simulink model "SF007A_SysFricLrng"  (R2013b)
settings: Solver=FixedStepDiscrete  SolverMode=SingleTasking  StartTime=0.0  StopTime=1  FixedStep=0.002  RelTol=1e-3
PostLoadFcn:
  | , if any(exist('dsrtsu_mdlpostloadfcn', 'file') == [2, 3, 6]), try dsrtsu_mdlpostloadfcn('Execute', bdroot); catch fprintf('Error in PostLoadFcn (dsrtsu_mdlpostloadfcn) for model "%s":\n %s\n', bdroot, lasterr); end, end,
undefined symbols (not defined in the file): ARCHGLBPRM_100MILLISEC_SEC_F32, ARCHGLBPRM_10MILLISEC_SEC_F32, ARCHGLBPRM_180OVERPI_ULS_F32, CONV100MICROSECTOSEC_ULS_F32, FLTINJ_SYSFRICLRNG_SYSFRICOFFS, FricLrngData, HiFricNtc, HWPTNUM_CNT_U08, HWPTNUMSUB1_CNT_U08, HWVELDECDIR_ULS_U08, HWVELINCDIR_ULS_U08, IDXCALCNSCAGFAC_ULS_U08, IDXSELN1_ULS_U08, IDXSELN2_ULS_U08, IDXSELN3_ULS_U08, LRNGENASCAFAC_MILLISEC_U32, NtcSts1, SCAGFACQUARTER_CNT_F32, SCAGFACTEN_CNT_U16, SECIDXSELN_ULS_U08, SysFricLrngBasLineEolFric, SysFricLrngBasLineFric, SysFricLrngBasLineHys, SysFricLrngBasLineRngCntr, SysFricLrngEolFricDifScagFac, SysFricLrngFricChgWght, SysFricLrngFricDiagcThd, SysFricLrngFricDiagcTiThd, SysFricLrngFricHysHwAgPt, SysFricLrngGain, SysFricLrngHwPosnAuthyThd, SysFricLrngHwVelConstrLim, SysFricLrngHwVelHiLim, SysFricLrngHwVelLoLim, SysFricLrngIgnCycFricChgLim, SysFricLrngLatAHiLim, SysFricLrngLatALoLim, SysFricLrngMaskVehSpd, SysFricLrngOperMod1, SysFricLrngRngCntrThd, SysFricLrngThd, SysFricLrngTHiLim, SysFricLrngTLoLim, SysFricLrngVehSpd, SYSFRICOFFSLIM_HWNWTMTR_F32, VEHSPDPTNUM1_ULS_U08, VEHSPDPTNUM2_ULS_U08
libraries: Fil x19, simulink x17, NxtrLim x10, NxtrAbslt x3, NxtrNvM x2, FixdToFloat x2, FloatToFixd x1, LnrIntrpn x1
(part 1 of 7)
settings Model: DSRTSU_INTERNAL_RTI_VER=370  DSRTSU_INTERNAL_RTI_TYPE=rti1401  Creator=fzv52m  LastModifiedBy=XZB1DB
settings Model: ModifiedHistory=|
  | Ver 004 Removed ignition latching of Friction Detection NTC to match software.
  | Limiting of P steps to one per ignition is being done with latching NTC allowing for the change
settings SolverCC: AutoInsertRateTranBlk=on  InsertRTBMode=Always
settings DataIOCC: LimitDataPoints=off  SaveFormat=Structure  ReturnWorkspaceOutputs=on
settings OptimizationCC: BlockReduction=off  InlineParams=on  ZeroExternalMemoryAtStartup=off  ZeroInternalMemoryAtStartup=off  OptimizeModelRefInitCode=on  LifeSpan=1
settings DebuggingCC: SignalInfNanChecking=error  SignalRangeChecking=warning  UnderspecifiedInitializationDetection=Simplified  SolverPrmCheckMsg=error  InheritedTsInSrcMsg=error  DiscreteInheritContinuousMsg=error  SingleTaskRateTransMsg=error  TasksWithSamePriorityMsg=error  SigSpecEnsureSampleTimeMsg=error  CheckMatrixSingularityMsg=error  ParameterUnderflowMsg=error  ParameterPrecisionLossMsg=error  ParameterTunabilityLossMsg=error  FixptConstUnderflowMsg=warning  FixptConstOverflowMsg=warning  VectorMatrixConversionMsg=error  SignalLabelMismatchMsg=error  UnconnectedInputMsg=error  UnconnectedOutputMsg=error  UnconnectedLineMsg=error  SFcnCompatibilityMsg=error  UniqueDataStoreMsg=warning  BusObjectLabelMismatch=error  RootOutportRequireBusObject=error  AssertControl=DisableAll  ModelReferenceIOMsg=error  ModelReferenceVersionMismatchMessage=warning  ModelReferenceIOMismatchMessage=error  ModelReferenceCSMismatchMessage=warning  ModelReferenceDataLoggingMessage=error  StateNameClashWarn=warning  StrictBusMsg=ErrorOnBusTreatedAsVector  NonBusSignalsTreatedAsBus=error  SFUnexpectedBacktrackingDiag=error  SFInvalidInputDataAccessInChartInitDiag=error  SFNoUnconditionalDefaultTransitionDiag=error  SFTransitionOutsideNaturalParentDiag=error  SFUnconditionalTransitionShadowingDiag=error  SFUndirectedBroadcastEventsDiag=error
settings ModelReferenceCC: ModelReferenceNumInstancesAllowed=Single
settings SFSimCC: SimGenImportedTypeDefs=on
settings RTWCC: SystemTargetFile=autosar.tlc  GenCodeOnly=on  TemplateMakefile=ert_default_tmf  Description=AUTOSAR  GenerateReport=on  ProcessScript=autosar_make_rtw_hook  LaunchReport=on
settings CodeAppCC: GenerateComments=off  IgnoreCustomStorageClasses=off  CustomSymbolStrType=$N$R$M  CustomSymbolStrBlkIO=$N$M  SimulinkBlockComments=off
settings STFCustomTargetCC: ParMdlRefBuildCompliant=on  CompOptLevelCompliant=on  IncludeMdlTerminateFcn=off  CombineOutputUpdateFcns=on  SuppressErrorStatus=on  ERTFirstTimeCompliant=on  ERTCustomFileBanners=on  SupportNonFinite=off  SupportComplex=off  SupportContinuousTime=off  SupportNonInlinedSFcns=off  MATLABClassNameForMDSCustomization=Simulink.SoftwareTarget.ERTCustomization  AutosarCompliant=on  GRTInterface=off  SystemTargetFile=autosar.tlc
settings ERTTargetCC: CodeReplacementLibrary=ANSI_C  ConcurrentExecutionCompliant=off  IncludeMdlTerminateFcn=off  SuppressErrorStatus=on  SupportNonFinite=off  SupportComplex=off  ModelStepFunctionPrototypeControlCompliant=off  CPPClassGenCompliant=off  AutosarCompliant=on  InlinedParameterPlacement=NonHierarchical  ERTCustomFileTemplate=example_file_process.tlc  EnableUserReplacementTypes=on

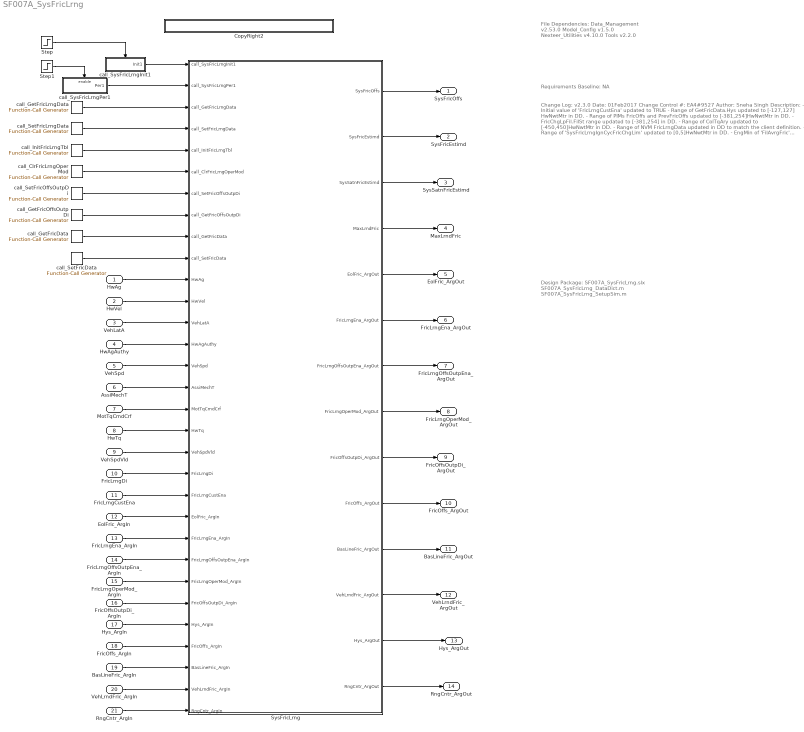
== system SF007A_SysFricLrng ==
  note: Requirements Baseline: NA
  note: File Dependencies:
      |
      | Data_Management v2.53.0
      | Model_Config v1.5.0
      | Nexteer_Utilities v4.10.0
      | Tools v2.2.0
  note: Change Log:
      |
      | v2.3.0
      | Date: 01Feb2017
      | Change Control #: EA4#9527
      | Author: Sneha Singh
      | Description:
      | - Initial value of 'FricLrngCustEna' updated to TRUE
      | - Range of GetFricData.Hys updated to [-127,127] HwNwtMtr in DD.
      | - Range of PIMs FricOffs and PrevFricOffs updated to [-381,254]HwNwtMtr in DD.
      | - FricChgLpFil.FilSt range updated to [-381,254] in DD.
      | - Range of ColTqAry updated to [-450,450]HwNwtMtr in DD.
      | - Range of NVM FricLrngData updated in DD to match the client definition.
      | - Range of 'SysFricLrngIgnCycFricChgLim' updated to [0,5]HwNwtMtr in DD.
      | - EngMin of 'FilAvrgFric' updated to -254 HwNwtMtr in DD.
      | - Range of 'SatnAvrgFric' updated to [-5,132]HwNwtMtr in DD.
      | - Definition of 'GetFricData' and 'SetFricData' updated in DD.
      | - Dimenions of NVM 'FricLrngData' updated in DD.
      | - Typecasting in the model has been updated to match source code.
      |
      | v2.2.0
      | Date: 29-NOV-2016
      | Change Control: EA4#8321
      | Function Owner:  Rangarajan Ramnujam
      | Description:
      | 1) Changes/clarification according to anomaly EA4#8103
      | 2) Added 'Get' and 'Set' client calls as per CR EA4#8418
      |
      |
      | v2.1.0
      | 1) Add output saturation for 'MaxLrndFric'
      | 2) Saturation constants added instead of using 'EngMin' and 'EngMax'
      |
      | v2.0.0
      | 1) Added extra output for Maximum Raw Average friction: Same friction value used for NTC diagnostic
      | 2)Else conditions added for LrngEna variable under path:
      | SF007A_SysFricLrng/SysFricLrng/SysFricLrngPer1/RunningAndCalibrationModes/RunningMode
      |
      | v1.4.0
      | 1) OR gate replaced with AND for LrngEna variable under path:
      | SF007A_SysFricLrng/SysFricLrng/SysFricLrngPer1/RunningAndCalibrationModes
      | 2) Logic updated under path
      | SF007A_SysFricLrng/SysFricLrng/SysFricLrngPer1/RunningAndCalibrationModes/Running Mode
      | 3) Eng min to -127 and Eng max to 254 updated for PIM 'FilAvrgFric' in Data Dict
      | 4) Logic for Indices calculation updated under below path. This change needed only in model as
      |     model uses one based Index logic. No code change required for this.
      |     SF007A_SysFricLrng/SysFricLrng/SysFricLrngPer1/RunningAndCalibrationModes/FricLearning/Indices Calculation
      | - Changes are highlighted in red. Code change needed for above mentioned changes 1, 2, and 4.
      |
      | v1.3.1
      | Date: 18-JULY-2016
      | Change Control: EA4#6450
      | DRW:  Hari Prasad(KPIT)
      | Description:
      | - Anomaly EA4#6361 Fixing for Gate variable look up table indexing.
      |   Removed 'Gate_Cnt_T_u08' temporary data store memory block.
      |   Logic related to it has been updated.
      | - Changes are highlighted in red. No code change needed.
      |
      | v1.3.0
      | Date: 07-APR-2016
      | Change Control #4835:
      | DRW:  Muragesh Asundi
      | Description:
      | - List of issues fixed are available under
      |   Doc/SF007_FDD_Issues.xlsx/Issues in V1.2.0
      | - In below path, Changed Gate from PIM to port inside subsystem
      |  as PIM wholds extra increment inside while loop
      |   SF007A_SysFricLrng/SysFricLrng/SysFricLrngPer1/RunningAndCalibrationModes/
      |   FricLearning/Range Counter Manager/Range Counter Control
      |
      | v1.2.0
      | Date: 30-Mar-2016
      | Change Control #4835:
      | DR W:  Muragesh Asundi
      | Description:
      | - List of issues fixed are available under
      |   Doc/SF007_FDD_Issues.xlsx/Issues in V1.1.0
      | - 'SetFricLrngOperMod' renamed to 'SetFricLrngData'
      | - 'SetEolFric' removed and merged with 'SetFricLrngData'
      | - Following PIMs have been removed from model and DD
      | 'HwAgPrev', 'HwVelPrev', 'ColTq'
      | - Monotony of callibration table 'SysFricLrngFricHysHwAgPt'
      | changed to 'Strictly_Increasing'
      | - Init value of PIM 'TotCntr' changed to 1
      |
      | v1.1.0
      | Date: 25-Mar-2016
      | Change Control #4835:
      | DRW:  Hari Prasad
      | Description:
      | - List of issues fixed are available under
      |   Doc/SF007_FDD_Issues.xlsx
      | - Changes are highlighed in red color
      |
      | v1.0.0
      | Date: 11-Mar-2016
      | Change Control #2719:
      | DRW:  Hari Prasad, Muragesh Asundi
      | Description:
      | - Initial Release of EA4 from EA3 V008
  note: Design Package:
      |
      | SF007A_SysFricLrng.slx
      | SF007A_SysFricLrng_DataDict.m
      | SF007A_SysFricLrng_SetupSim.m
  HwAg : Inport
  HwVel : Inport  Port=2
  VehLatA : Inport  Port=3
  HwAgAuthy : Inport  Port=4
  VehSpd : Inport  Port=5
  AssiMechT : Inport  Port=6
  MotTqCmdCrf : Inport  Port=7
  HwTq : Inport  Port=8
  VehSpdVld : Inport  Port=9
  FricLrngDi : Inport  Port=10
  FricLrngCustEna : Inport  Port=11
  EolFric_ArgIn : Inport  Port=12
  FricLrngEna_ArgIn : Inport  Port=13
  FricLrngOffsOutpEna_ArgIn : Inport  Port=14
  FricLrngOperMod_ArgIn : Inport  Port=15
  FricOffsOutpDi_ArgIn : Inport  Port=16
  Hys_ArgIn : Inport  Port=17
  FricOffs_ArgIn : Inport  Port=18
  BasLineFric_ArgIn : Inport  Port=19
  VehLrndFric_ArgIn : Inport  Port=20
  RngCntr_ArgIn : Inport  Port=21
  CopyRight2 : Subsystem  Description=|  mask(Copyright Information){none=on}
      | Copyright info block.                                               
      |                                                                     
      | Place copyright information at the top of every subsystem in design.
      mask prompts: none "No parameters"
      mask help: Place copyright information at the top of every subsystem in design.
      mask Display:
      | NxtrConf = 'Nexteer Confidential';
      | 
      | sys = bdroot; %handle for the current model ("system")
      | first = get_param(sys,'Created');
      | first = first(end-3:end);  %year is last four digits
      | 
      | last = get_param(sys,'LastModifiedDate');
      | if isempty(last)
      |     last = datestr(now,'yyyy');
      | else
      |     last = last(end-3:end);
      | end
      | 
      | if strcmp(first,last)
      |     fprintf('%s -- Copyright %s Nexteer',NxtrConf,first)
      | else
      |     fprintf('%s -- %s%s- %s Nexteer',NxtrConf,char(169),first,last)
      | end
  Step : Step  Before=1  After=0  SampleTime=0.010
  Step1 : Step  SampleTime=0.010
  SysFricLrng : Subsystem
  call_ClrFricLrngOperMod : simulink/Ports & Subsystems/Function-Call Generator  sample_time=0.010  numberOfIterations=1
  call_GetFricData : simulink/Ports & Subsystems/Function-Call Generator  sample_time=0.010  numberOfIterations=1
  call_GetFricLrngData : simulink/Ports & Subsystems/Function-Call Generator  sample_time=0.010  numberOfIterations=1
  call_GetFricOffsOutpDi : simulink/Ports & Subsystems/Function-Call Generator  sample_time=0.010  numberOfIterations=1
  call_InitFricLrngTbl : simulink/Ports & Subsystems/Function-Call Generator  sample_time=0.010  numberOfIterations=1
  call_SetFricData : simulink/Ports & Subsystems/Function-Call Generator  sample_time=0.010  numberOfIterations=1
  call_SetFricLrngData : simulink/Ports & Subsystems/Function-Call Generator  sample_time=0.010  numberOfIterations=1
  call_SetFricOffsOutpDi : simulink/Ports & Subsystems/Function-Call Generator  sample_time=0.010  numberOfIterations=1
  call_SysFricLrngInit1 : Subsystem  TreatAsAtomicUnit=on
  call_SysFricLrngPer1 : Subsystem  TreatAsAtomicUnit=on
  SysFricOffs : Outport
  SysFricEstimd : Outport  Port=2
  SysSatnFricEstimd : Outport  Port=3
  MaxLrndFric : Outport  Port=4
  EolFric_ArgOut : Outport  Port=5
  FricLrngEna_ArgOut : Outport  Port=6
  FricLrngOffsOutpEna_ArgOut : Outport  Port=7
  FricLrngOperMod_ArgOut : Outport  Port=8
  FricOffsOutpDi_ArgOut : Outport  Port=9
  FricOffs_ArgOut : Outport  Port=10
  BasLineFric_ArgOut : Outport  Port=11
  VehLrndFric_ArgOut : Outport  Port=12
  Hys_ArgOut : Outport  Port=13
  RngCntr_ArgOut : Outport  Port=14
  wires:
  MotTqCmdCrf/1 -> SysFricLrng/17(MotTqCmdCrf)
  FricLrngDi/1 -> SysFricLrng/20(FricLrngDi)
  HwVel/1 -> SysFricLrng/12(HwVel)
  HwAg/1 -> SysFricLrng/11(HwAg)
  HwTq/1 -> SysFricLrng/18(HwTq)
  VehSpdVld/1 -> SysFricLrng/19(VehSpdVld)
  call_GetFricLrngData/1 -> SysFricLrng/3(call_GetFricLrngData)
  HwAgAuthy/1 -> SysFricLrng/14(HwAgAuthy)
  AssiMechT/1 -> SysFricLrng/16(AssiMechT)
  VehLatA/1 -> SysFricLrng/13(VehLatA)
  VehSpd/1 -> SysFricLrng/15(VehSpd)
  SysFricLrng/1(SysFricOffs) -> SysFricOffs/1
  SysFricLrng/3(SysSatnFricEstimd) -> SysSatnFricEstimd/1
  SysFricLrng/2(SysFricEstimd) -> SysFricEstimd/1
  FricLrngCustEna/1 -> SysFricLrng/21(FricLrngCustEna)
  call_SetFricLrngData/1 -> SysFricLrng/4(call_SetFricLrngData)
  call_InitFricLrngTbl/1 -> SysFricLrng/5(call_InitFricLrngTbl)
  call_SetFricOffsOutpDi/1 -> SysFricLrng/7(call_SetFricOffsOutpDi)
  call_GetFricOffsOutpDi/1 -> SysFricLrng/8(call_GetFricOffsOutpDi)
  call_ClrFricLrngOperMod/1 -> SysFricLrng/6(call_ClrFricLrngOperMod)
  SysFricLrng/6(FricLrngEna_ArgOut) -> FricLrngEna_ArgOut/1
  SysFricLrng/8(FricLrngOperMod_ArgOut) -> FricLrngOperMod_ArgOut/1
  SysFricLrng/7(FricLrngOffsOutpEna_ArgOut) -> FricLrngOffsOutpEna_ArgOut/1
  SysFricLrng/9(FricOffsOutpDi_ArgOut) -> FricOffsOutpDi_ArgOut/1
  SysFricLrng/5(EolFric_ArgOut) -> EolFric_ArgOut/1
  FricLrngEna_ArgIn/1 -> SysFricLrng/23(FricLrngEna_ArgIn)
  FricLrngOffsOutpEna_ArgIn/1 -> SysFricLrng/24(FricLrngOffsOutpEna_ArgIn)
  FricLrngOperMod_ArgIn/1 -> SysFricLrng/25(FricLrngOperMod_ArgIn)
  EolFric_ArgIn/1 -> SysFricLrng/22(EolFric_ArgIn)
  FricOffsOutpDi_ArgIn/1 -> SysFricLrng/26(FricOffsOutpDi_ArgIn)
  call_SysFricLrngInit1/1(Init1) -> SysFricLrng/1(call_SysFricLrngInit1)
  Step/1 -> call_SysFricLrngInit1/Enable
  call_SysFricLrngPer1/1(Per1) -> SysFricLrng/2(call_SysFricLrngPer1)
  Step1/1 -> call_SysFricLrngPer1/Enable
  SysFricLrng/4(MaxLrndFric) -> MaxLrndFric/1
  SysFricLrng/10(FricOffs_ArgOut) -> FricOffs_ArgOut/1
  SysFricLrng/13(Hys_ArgOut) -> Hys_ArgOut/1
  SysFricLrng/11(BasLineFric_ArgOut) -> BasLineFric_ArgOut/1
  SysFricLrng/14(RngCntr_ArgOut) -> RngCntr_ArgOut/1
  SysFricLrng/12(VehLrndFric_ArgOut) -> VehLrndFric_ArgOut/1
  call_SetFricData/1 -> SysFricLrng/10(call_SetFricData)
  call_GetFricData/1 -> SysFricLrng/9(call_GetFricData)
  FricOffs_ArgIn/1 -> SysFricLrng/28(FricOffs_ArgIn)
  VehLrndFric_ArgIn/1 -> SysFricLrng/30(VehLrndFric_ArgIn)
  BasLineFric_ArgIn/1 -> SysFricLrng/29(BasLineFric_ArgIn)
  RngCntr_ArgIn/1 -> SysFricLrng/31(RngCntr_ArgIn)
  Hys_ArgIn/1 -> SysFricLrng/27(Hys_ArgIn)

== system SF007A_SysFricLrng/CopyRight2 ==

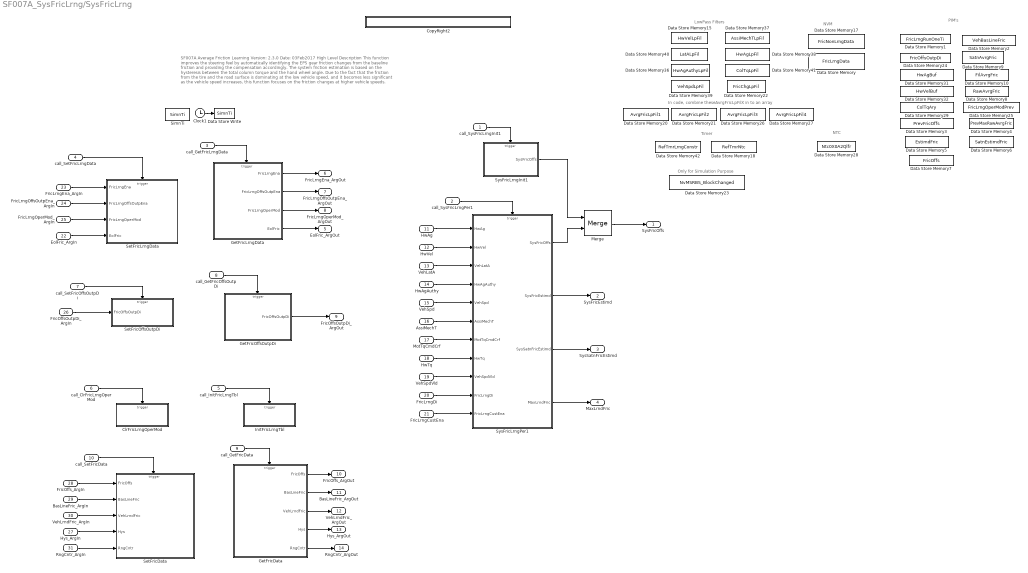
== system SF007A_SysFricLrng/SysFricLrng ==
  note: In code, combine theseAvrgFricLpFilX in to an array
  note: Only for Simulation Purpose
  note: PIM's
  note: Timer
  note: LowPass Filters
  note: NVM
  note: SF007A  Average Friction Learning
      | Version: 2.3.0          																															 					Date: 03Feb2017
      |
      | High Level Description
      |
      | This function improves the steering feel by automatically identifying the EPS gear friction changes from the baseline friction and providing the compensation accordingly. The system friction estimation
      |  is based on the hysteresis between the total column torque and the hand wheel angle. Due to the fact that the friction from the tire and the road surface is dominating at the low vehicle speed,  and it
      | becomes less significant as the vehicle speed increases, this function focuses on the friction changes at higher vehicle speeds.
  note: NTC
  call_SysFricLrngInit1 : Inport
  call_SysFricLrngPer1 : Inport  Port=2
  call_GetFricLrngData : Inport  Port=3
  call_SetFricLrngData : Inport  Port=4
  call_InitFricLrngTbl : Inport  Port=5
  call_ClrFricLrngOperMod : Inport  Port=6
  call_SetFricOffsOutpDi : Inport  Port=7
  call_GetFricOffsOutpDi : Inport  Port=8
  call_GetFricData : Inport  Port=9
  call_SetFricData : Inport  Port=10
  HwAg : Inport  Port=11
  HwVel : Inport  Port=12
  VehLatA : Inport  Port=13
  HwAgAuthy : Inport  Port=14
  VehSpd : Inport  Port=15
  AssiMechT : Inport  Port=16
  MotTqCmdCrf : Inport  Port=17
  HwTq : Inport  Port=18
  VehSpdVld : Inport  Port=19
  FricLrngDi : Inport  Port=20
  FricLrngCustEna : Inport  Port=21
  EolFric_ArgIn : Inport  Port=22
  FricLrngEna_ArgIn : Inport  Port=23
  FricLrngOffsOutpEna_ArgIn : Inport  Port=24
  FricLrngOperMod_ArgIn : Inport  Port=25
  FricOffsOutpDi_ArgIn : Inport  Port=26
  Hys_ArgIn : Inport  Port=27
  FricOffs_ArgIn : Inport  Port=28
  BasLineFric_ArgIn : Inport  Port=29
  VehLrndFric_ArgIn : Inport  Port=30
  RngCntr_ArgIn : Inport  Port=31
  Clock1 : Clock
  ClrFricLrngOperMod : Subsystem
  CopyRight2 : Subsystem  Description=|  mask(Copyright Information){none=on}
      | Copyright info block.                                               
      |                                                                     
      | Place copyright information at the top of every subsystem in design.
      mask prompts: none "No parameters"
      mask help: Place copyright information at the top of every subsystem in design.
      mask Display:
      | NxtrConf = 'Nexteer Confidential';
      | 
      | sys = bdroot; %handle for the current model ("system")
      | first = get_param(sys,'Created');
      | if(isempty(first))
      |     first = datestr(now,'yyyy');
      | else
      |     first = first(end-3:end);  %year is last four digits
      | end
      | 
      | last = get_param(sys,'LastModifiedDate');
      | if isempty(last)
      |     last = datestr(now,'yyyy');
      | else
      |     last = last(end-3:end);
      | end
      | 
      | if strcmp(first,last)
      |     fprintf('%s -- Copyright %s Nexteer',NxtrConf,first)
      | else
      |     fprintf('%s -- %s%s- %s Nexteer',NxtrConf,char(169),first,last)
      | end
  Data Store Memory : DataStoreMemory  DataStoreName=FricLrngData  InitialValue=[]  OutDataTypeStr=Bus: SysFricDataRec1  StateMustResolveToSignalObject=on
  Data Store Memory1 : DataStoreMemory  DataStoreName=FricLrngRunOneTi  StateMustResolveToSignalObject=on
  Data Store Memory10 : DataStoreMemory  DataStoreName=FilAvrgFric  InitialValue=[0 0 0 0]  OutDataTypeStr=single  StateMustResolveToSignalObject=on
  Data Store Memory15 : DataStoreMemory  DataStoreName=HwVelLpFil  InitialValue=struct('FilSt',single(0),'FilGain',single(0))  OutDataTypeStr=Bus: FilLpRec1  StateMustResolveToSignalObject=on
  Data Store Memory17 : DataStoreMemory  DataStoreName=FricNonLrngData  InitialValue=[]  OutDataTypeStr=Bus: SysFricNonLrngDataRec1  StateMustResolveToSignalObject=on
  Data Store Memory18 : DataStoreMemory  DataStoreName=RefTmrNtc  StateMustResolveToSignalObject=on
  Data Store Memory2 : DataStoreMemory  DataStoreName=VehBasLineFric  InitialValue=[0 0 0 0]  StateMustResolveToSignalObject=on
  Data Store Memory20 : DataStoreMemory  DataStoreName=AvrgFricLpFil1  InitialValue=struct('FilSt',single(0),'FilGain',single(0))  OutDataTypeStr=Bus: FilLpRec1  StateMustResolveToSignalObject=on
  Data Store Memory21 : DataStoreMemory  DataStoreName=AvrgFricLpFil2  InitialValue=struct('FilSt',single(0),'FilGain',single(0))  OutDataTypeStr=Bus: FilLpRec1  StateMustResolveToSignalObject=on
  Data Store Memory22 : DataStoreMemory  DataStoreName=FricChgLpFil  InitialValue=struct('FilSt',single(0),'FilGain',single(0))  OutDataTypeStr=Bus: FilLpRec1  StateMustResolveToSignalObject=on
  Data Store Memory23 : DataStoreMemory  DataStoreName=NvMSRBS_BlockChanged
  Data Store Memory24 : DataStoreMemory  DataStoreName=FricOffsOutpDi  StateMustResolveToSignalObject=on
  Data Store Memory25 : DataStoreMemory  DataStoreName=FricLrngOperModPrev  InitialValue=[]  StateMustResolveToSignalObject=on
  Data Store Memory26 : DataStoreMemory  DataStoreName=AvrgFricLpFil3  InitialValue=struct('FilSt',single(0),'FilGain',single(0))  OutDataTypeStr=Bus: FilLpRec1  StateMustResolveToSignalObject=on
  Data Store Memory27 : DataStoreMemory  DataStoreName=AvrgFricLpFil4  InitialValue=struct('FilSt',single(0),'FilGain',single(0))  OutDataTypeStr=Bus: FilLpRec1  StateMustResolveToSignalObject=on
  Data Store Memory28 : DataStoreMemory  DataStoreName=Ntc0X0A2Qlfr  InitialValue=SigQlfr1.SIGQLFR_NORES
  Data Store Memory29 : DataStoreMemory  DataStoreName=ColTqAry  InitialValue=[]  StateMustResolveToSignalObject=on
  Data Store Memory3 : DataStoreMemory  DataStoreName=PrevFricOffs  InitialValue=[]  StateMustResolveToSignalObject=on
  Data Store Memory31 : DataStoreMemory  DataStoreName=HwAgBuf  InitialValue=[0 0 0 0 0 0 0 0 0 0 0 0]  StateMustResolveToSignalObject=on
  Data Store Memory32 : DataStoreMemory  DataStoreName=HwVelBuf  InitialValue=[0 0 0 0 0 0 0 0 0 0 0 0]  StateMustResolveToSignalObject=on
  Data Store Memory36 : DataStoreMemory  DataStoreName=HwAgAuthyLpFil  InitialValue=struct('FilSt',single(0),'FilGain',single(0))  OutDataTypeStr=Bus: FilLpRec1  StateMustResolveToSignalObject=on
  Data Store Memory37 : DataStoreMemory  DataStoreName=AssiMechTLpFil  InitialValue=struct('FilSt',single(0),'FilGain',single(0))  OutDataTypeStr=Bus: FilLpRec1  StateMustResolveToSignalObject=on
  Data Store Memory38 : DataStoreMemory  DataStoreName=HwAgLpFil  InitialValue=struct('FilSt',single(0),'FilGain',single(0))  OutDataTypeStr=Bus: FilLpRec1  StateMustResolveToSignalObject=on
  Data Store Memory39 : DataStoreMemory  DataStoreName=VehSpdLpFil  InitialValue=struct('FilSt',single(0),'FilGain',single(0))  OutDataTypeStr=Bus: FilLpRec1  StateMustResolveToSignalObject=on
  Data Store Memory4 : DataStoreMemory  DataStoreName=PrevMaxRawAvrgFric  InitialValue=[]  OutDataTypeStr=single  StateMustResolveToSignalObject=on
  Data Store Memory40 : DataStoreMemory  DataStoreName=LatALpFil  InitialValue=struct('FilSt',single(0),'FilGain',single(0))  OutDataTypeStr=Bus: FilLpRec1  StateMustResolveToSignalObject=on
  Data Store Memory41 : DataStoreMemory  DataStoreName=ColTqLpFil  InitialValue=struct('FilSt',single(0),'FilGain',single(0))  OutDataTypeStr=Bus: FilLpRec1  StateMustResolveToSignalObject=on
  Data Store Memory42 : DataStoreMemory  DataStoreName=RefTmrLrngConstr  StateMustResolveToSignalObject=on
  Data Store Memory5 : DataStoreMemory  DataStoreName=EstimdFric  InitialValue=[]  OutDataTypeStr=single  StateMustResolveToSignalObject=on
  Data Store Memory6 : DataStoreMemory  DataStoreName=SatnEstimdFric  InitialValue=[]  OutDataTypeStr=single  StateMustResolveToSignalObject=on
  Data Store Memory7 : DataStoreMemory  DataStoreName=FricOffs  InitialValue=[]  OutDataTypeStr=single  StateMustResolveToSignalObject=on
  Data Store Memory8 : DataStoreMemory  DataStoreName=RawAvrgFric  InitialValue=[0 0 0 0]  OutDataTypeStr=single  StateMustResolveToSignalObject=on
  Data Store Memory9 : DataStoreMemory  DataStoreName=SatnAvrgFric  InitialValue=[0 0 0 0]  StateMustResolveToSignalObject=on
  Data Store Write : DataStoreWrite  DataStoreName=SimnTi
  GetFricData : Subsystem
  GetFricLrngData : Subsystem
  GetFricOffsOutpDi : Subsystem
  InitFricLrngTbl : Subsystem
  Merge : Merge
  SetFricData : Subsystem
  SetFricLrngData : Subsystem
  SetFricOffsOutpDi : Subsystem
  SimnTi : DataStoreMemory  DataStoreName=SimnTi
  SysFricLrngInit1 : Subsystem
  SysFricLrngPer1 : Subsystem
  SysFricOffs : Outport
  SysFricEstimd : Outport  Port=2
  SysSatnFricEstimd : Outport  Port=3
  MaxLrndFric : Outport  Port=4
  EolFric_ArgOut : Outport  Port=5
  FricLrngEna_ArgOut : Outport  Port=6
  FricLrngOffsOutpEna_ArgOut : Outport  Port=7
  FricLrngOperMod_ArgOut : Outport  Port=8
  FricOffsOutpDi_ArgOut : Outport  Port=9
  FricOffs_ArgOut : Outport  Port=10
  BasLineFric_ArgOut : Outport  Port=11
  VehLrndFric_ArgOut : Outport  Port=12
  Hys_ArgOut : Outport  Port=13
  RngCntr_ArgOut : Outport  Port=14
  wires:
  call_SysFricLrngInit1/1 -> SysFricLrngInit1/Trigger
  HwAg/1 -> SysFricLrngPer1/1(HwAg)
  HwVel/1 -> SysFricLrngPer1/2(HwVel)
  VehLatA/1 -> SysFricLrngPer1/3(VehLatA)
  HwAgAuthy/1 -> SysFricLrngPer1/4(HwAgAuthy)
  VehSpd/1 -> SysFricLrngPer1/5(VehSpd)
  AssiMechT/1 -> SysFricLrngPer1/6(AssiMechT)
  MotTqCmdCrf/1 -> SysFricLrngPer1/7(MotTqCmdCrf)
  HwTq/1 -> SysFricLrngPer1/8(HwTq)
  VehSpdVld/1 -> SysFricLrngPer1/9(VehSpdVld)
  FricLrngDi/1 -> SysFricLrngPer1/10(FricLrngDi)
  call_SysFricLrngPer1/1 -> SysFricLrngPer1/Trigger
  Clock1/1 -> Data Store Write/1
  SysFricLrngPer1/3(SysSatnFricEstimd) -> SysSatnFricEstimd/1
  SysFricLrngPer1/2(SysFricEstimd) -> SysFricEstimd/1
  FricLrngCustEna/1 -> SysFricLrngPer1/11(FricLrngCustEna)
  call_SetFricLrngData/1 -> SetFricLrngData/Trigger
  call_GetFricLrngData/1 -> GetFricLrngData/Trigger
  call_SetFricOffsOutpDi/1 -> SetFricOffsOutpDi/Trigger
  call_GetFricOffsOutpDi/1 -> GetFricOffsOutpDi/Trigger
  call_InitFricLrngTbl/1 -> InitFricLrngTbl/Trigger
  call_ClrFricLrngOperMod/1 -> ClrFricLrngOperMod/Trigger
  GetFricLrngData/1(FricLrngEna) -> FricLrngEna_ArgOut/1
  GetFricLrngData/3(FricLrngOperMod) -> FricLrngOperMod_ArgOut/1
  GetFricLrngData/2(FricLrngOffsOutpEna) -> FricLrngOffsOutpEna_ArgOut/1
  FricLrngEna_ArgIn/1 -> SetFricLrngData/1(FricLrngEna)
  FricLrngOperMod_ArgIn/1 -> SetFricLrngData/3(FricLrngOperMod)
  FricLrngOffsOutpEna_ArgIn/1 -> SetFricLrngData/2(FricLrngOffsOutpEna)
  FricOffsOutpDi_ArgIn/1 -> SetFricOffsOutpDi/1(FricOffsOutpDi)
  GetFricOffsOutpDi/1(FricOffsOutpDi) -> FricOffsOutpDi_ArgOut/1
  GetFricLrngData/4(EolFric) -> EolFric_ArgOut/1
  SysFricLrngInit1/1(SysFricOffs) -> Merge/1
  SysFricLrngPer1/1(SysFricOffs) -> Merge/2
  Merge/1 -> SysFricOffs/1
  EolFric_ArgIn/1 -> SetFricLrngData/4(EolFric)
  SysFricLrngPer1/4(MaxLrndFric) -> MaxLrndFric/1
  call_SetFricData/1 -> SetFricData/Trigger
  call_GetFricData/1 -> GetFricData/Trigger
  FricOffs_ArgIn/1 -> SetFricData/1(FricOffs)
  VehLrndFric_ArgIn/1 -> SetFricData/3(VehLrndFric)
  BasLineFric_ArgIn/1 -> SetFricData/2(BasLineFric)
  RngCntr_ArgIn/1 -> SetFricData/5(RngCntr)
  GetFricData/1(FricOffs) -> FricOffs_ArgOut/1
  GetFricData/4(Hys) -> Hys_ArgOut/1
  GetFricData/2(BasLineFric) -> BasLineFric_ArgOut/1
  GetFricData/5(RngCntr) -> RngCntr_ArgOut/1
  GetFricData/3(VehLrndFric) -> VehLrndFric_ArgOut/1
  Hys_ArgIn/1 -> SetFricData/4(Hys)

== system SF007A_SysFricLrng/call_SysFricLrngInit1 ==
  Enable : EnablePort
  CopyRight2 : Subsystem  Description=|  mask(Copyright Information){none=on}
      | Copyright info block.                                               
      |                                                                     
      | Place copyright information at the top of every subsystem in design.
      mask prompts: none "No parameters"
      mask help: Place copyright information at the top of every subsystem in design.
      mask Display:
      | NxtrConf = 'Nexteer Confidential';
      | 
      | sys = bdroot; %handle for the current model ("system")
      | first = get_param(sys,'Created');
      | if(isempty(first))
      |     first = datestr(now,'yyyy');
      | else
      |     first = first(end-3:end);  %year is last four digits
      | end
      | 
      | last = get_param(sys,'LastModifiedDate');
      | if isempty(last)
      |     last = datestr(now,'yyyy');
      | else
      |     last = last(end-3:end);
      | end
      | 
      | if strcmp(first,last)
      |     fprintf('%s -- Copyright %s Nexteer',NxtrConf,first)
      | else
      |     fprintf('%s -- %s%s- %s Nexteer',NxtrConf,char(169),first,last)
      | end
  Function-Call Generator : simulink/Ports & Subsystems/Function-Call Generator  sample_time=.01  numberOfIterations=1
  Init1 : Outport
  wires:
  Function-Call Generator/1 -> Init1/1

== system SF007A_SysFricLrng/call_SysFricLrngPer1 ==
  Enable : EnablePort
  CopyRight2 : Subsystem  Description=|  mask(Copyright Information){none=on}
      | Copyright info block.                                               
      |                                                                     
      | Place copyright information at the top of every subsystem in design.
      mask prompts: none "No parameters"
      mask help: Place copyright information at the top of every subsystem in design.
      mask Display:
      | NxtrConf = 'Nexteer Confidential';
      | 
      | sys = bdroot; %handle for the current model ("system")
      | first = get_param(sys,'Created');
      | if(isempty(first))
      |     first = datestr(now,'yyyy');
      | else
      |     first = first(end-3:end);  %year is last four digits
      | end
      | 
      | last = get_param(sys,'LastModifiedDate');
      | if isempty(last)
      |     last = datestr(now,'yyyy');
      | else
      |     last = last(end-3:end);
      | end
      | 
      | if strcmp(first,last)
      |     fprintf('%s -- Copyright %s Nexteer',NxtrConf,first)
      | else
      |     fprintf('%s -- %s%s- %s Nexteer',NxtrConf,char(169),first,last)
      | end
  Function-Call Generator : simulink/Ports & Subsystems/Function-Call Generator  sample_time=.01  numberOfIterations=1
  Per1 : Outport
  wires:
  Function-Call Generator/1 -> Per1/1

== system SF007A_SysFricLrng/SysFricLrng/ClrFricLrngOperMod ==
  note: Set Ram Block Status for 'FricLrngData' moved to Init
  function : TriggerPort  TriggerType=function-call
  Constant1 : Constant  Value=false  OutDataTypeStr=boolean
      settings: AttributesFormatString=%<OutDataTypeStr>
  CopyRight2 : Subsystem  Description=|  mask(Copyright Information){none=on}
      | Copyright info block.                                               
      |                                                                     
      | Place copyright information at the top of every subsystem in design.
      mask prompts: none "No parameters"
      mask help: Place copyright information at the top of every subsystem in design.
      mask Display:
      | NxtrConf = 'Nexteer Confidential';
      | 
      | sys = bdroot; %handle for the current model ("system")
      | first = get_param(sys,'Created');
      | if(isempty(first))
      |     first = datestr(now,'yyyy');
      | else
      |     first = first(end-3:end);  %year is last four digits
      | end
      | 
      | last = get_param(sys,'LastModifiedDate');
      | if isempty(last)
      |     last = datestr(now,'yyyy');
      | else
      |     last = last(end-3:end);
      | end
      | 
      | if strcmp(first,last)
      |     fprintf('%s -- Copyright %s Nexteer',NxtrConf,first)
      | else
      |     fprintf('%s -- %s%s- %s Nexteer',NxtrConf,char(169),first,last)
      | end
  Data Store Read : DataStoreRead  DataStoreName=FricLrngData  DataStoreElements=FricLrngData.SysFricLrngOperMod
  Data Store Write : DataStoreWrite  DataStoreName=FricLrngOperModPrev
  Data Store Write1 : DataStoreWrite  DataStoreName=FricLrngData  DataStoreElements=FricLrngData.SysFricLrngOperMod
  Data Store Write2 : DataStoreWrite  DataStoreName=FricLrngRunOneTi
  Enumerated Constant : simulink/Sources/Enumerated Constant  OutDataTypeStr=Enum: SysFricLrngOperMod1  Value=SysFricLrngOperMod1.SYSFRICLRNGOPERMOD_CLEAR  SampleTime=inf
  wires:
  Constant1/1 -> Data Store Write2/1
  Enumerated Constant/1 -> Data Store Write1/1
  Data Store Read/1 -> Data Store Write/1

== system SF007A_SysFricLrng/SysFricLrng/CopyRight2 ==

== system SF007A_SysFricLrng/SysFricLrng/GetFricData ==
  note: Get NVM Data
  function : TriggerPort  TriggerType=function-call
  CopyRight2 : Subsystem  Description=|  mask(Copyright Information){none=on}
      | Copyright info block.                                               
      |                                                                     
      | Place copyright information at the top of every subsystem in design.
      mask prompts: none "No parameters"
      mask help: Place copyright information at the top of every subsystem in design.
      mask Display:
      | NxtrConf = 'Nexteer Confidential';
      | 
      | sys = bdroot; %handle for the current model ("system")
      | first = get_param(sys,'Created');
      | first = first(end-3:end);  %year is last four digits
      | 
      | last = get_param(sys,'LastModifiedDate');
      | if isempty(last)
      |     last = datestr(now,'yyyy');
      | else
      |     last = last(end-3:end);
      | end
      | 
      | if strcmp(first,last)
      |     fprintf('%s -- Copyright %s Nexteer',NxtrConf,first)
      | else
      |     fprintf('%s -- %s%s- %s Nexteer',NxtrConf,char(169),first,last)
      | end
  Data Store Read : DataStoreRead  DataStoreName=FricLrngData  DataStoreElements=FricLrngData.FricOffs#FricLrngData.BasLineFric(:,:)#FricLrngData.VehLrndFric(:,:)#FricLrngData.Hys(:,:)#FricLrngData.RngCntr(:,:)
  FricOffs : Outport
  BasLineFric : Outport  Port=2
  VehLrndFric : Outport  Port=3
  Hys : Outport  Port=4
  RngCntr : Outport  Port=5
  wires:
  Data Store Read/5 -> RngCntr/1
  Data Store Read/1 -> FricOffs/1
  Data Store Read/2 -> BasLineFric/1
  Data Store Read/3 -> VehLrndFric/1
  Data Store Read/4 -> Hys/1

== system SF007A_SysFricLrng/SysFricLrng/GetFricLrngData ==
  note: Get NVM Data
  function : TriggerPort  TriggerType=function-call
  CopyRight2 : Subsystem  Description=|  mask(Copyright Information){none=on}
      | Copyright info block.                                               
      |                                                                     
      | Place copyright information at the top of every subsystem in design.
      mask prompts: none "No parameters"
      mask help: Place copyright information at the top of every subsystem in design.
      mask Display:
      | NxtrConf = 'Nexteer Confidential';
      | 
      | sys = bdroot; %handle for the current model ("system")
      | first = get_param(sys,'Created');
      | first = first(end-3:end);  %year is last four digits
      | 
      | last = get_param(sys,'LastModifiedDate');
      | if isempty(last)
      |     last = datestr(now,'yyyy');
      | else
      |     last = last(end-3:end);
      | end
      | 
      | if strcmp(first,last)
      |     fprintf('%s -- Copyright %s Nexteer',NxtrConf,first)
      | else
      |     fprintf('%s -- %s%s- %s Nexteer',NxtrConf,char(169),first,last)
      | end
  Data Store Read : DataStoreRead  DataStoreName=FricLrngData  DataStoreElements=FricLrngData.SysFricLrngOperMod
  Data Store Read1 : DataStoreRead  DataStoreName=FricNonLrngData  DataStoreElements=FricNonLrngData.EnaFricLrng#FricNonLrngData.EnaFricOffsOutp#FricNonLrngData.EolFric
  FricLrngEna : Outport
  FricLrngOffsOutpEna : Outport  Port=2
  FricLrngOperMod : Outport  Port=3
  EolFric : Outport  Port=4
  wires:
  Data Store Read/1 -> FricLrngOperMod/1
  Data Store Read1/1 -> FricLrngEna/1
  Data Store Read1/2 -> FricLrngOffsOutpEna/1
  Data Store Read1/3 -> EolFric/1

== system SF007A_SysFricLrng/SysFricLrng/GetFricOffsOutpDi ==
  function : TriggerPort  TriggerType=function-call
  CopyRight2 : Subsystem  Description=|  mask(Copyright Information){none=on}
      | Copyright info block.                                               
      |                                                                     
      | Place copyright information at the top of every subsystem in design.
      mask prompts: none "No parameters"
      mask help: Place copyright information at the top of every subsystem in design.
      mask Display:
      | NxtrConf = 'Nexteer Confidential';
      | 
      | sys = bdroot; %handle for the current model ("system")
      | first = get_param(sys,'Created');
      | first = first(end-3:end);  %year is last four digits
      | 
      | last = get_param(sys,'LastModifiedDate');
      | if isempty(last)
      |     last = datestr(now,'yyyy');
      | else
      |     last = last(end-3:end);
      | end
      | 
      | if strcmp(first,last)
      |     fprintf('%s -- Copyright %s Nexteer',NxtrConf,first)
      | else
      |     fprintf('%s -- %s%s- %s Nexteer',NxtrConf,char(169),first,last)
      | end
  Data Store Read1 : DataStoreRead  DataStoreName=FricOffsOutpDi
  FricOffsOutpDi : Outport
  wires:
  Data Store Read1/1 -> FricOffsOutpDi/1

== system SF007A_SysFricLrng/SysFricLrng/InitFricLrngTbl ==
  note: Set Ram Block Status moved to Init
  function : TriggerPort  TriggerType=function-call
  Constant1 : Constant  Value=false  OutDataTypeStr=boolean
      settings: AttributesFormatString=%<OutDataTypeStr>
  CopyRight2 : Subsystem  Description=|  mask(Copyright Information){none=on}
      | Copyright info block.                                               
      |                                                                     
      | Place copyright information at the top of every subsystem in design.
      mask prompts: none "No parameters"
      mask help: Place copyright information at the top of every subsystem in design.
      mask Display:
      | NxtrConf = 'Nexteer Confidential';
      | 
      | sys = bdroot; %handle for the current model ("system")
      | first = get_param(sys,'Created');
      | if(isempty(first))
      |     first = datestr(now,'yyyy');
      | else
      |     first = first(end-3:end);  %year is last four digits
      | end
      | 
      | last = get_param(sys,'LastModifiedDate');
      | if isempty(last)
      |     last = datestr(now,'yyyy');
      | else
      |     last = last(end-3:end);
      | end
      | 
      | if strcmp(first,last)
      |     fprintf('%s -- Copyright %s Nexteer',NxtrConf,first)
      | else
      |     fprintf('%s -- %s%s- %s Nexteer',NxtrConf,char(169),first,last)
      | end
  Data Store Read : DataStoreRead  DataStoreName=FricLrngData  DataStoreElements=FricLrngData.SysFricLrngOperMod
  Data Store Write : DataStoreWrite  DataStoreName=FricLrngOperModPrev
  Data Store Write1 : DataStoreWrite  DataStoreName=FricLrngData  DataStoreElements=FricLrngData.SysFricLrngOperMod
  Data Store Write2 : DataStoreWrite  DataStoreName=FricLrngRunOneTi
  Enumerated Constant : simulink/Sources/Enumerated Constant  OutDataTypeStr=Enum: SysFricLrngOperMod1  Value=SysFricLrngOperMod1.SYSFRICLRNGOPERMOD_BASELINE  SampleTime=inf
  wires:
  Data Store Read/1 -> Data Store Write/1
  Enumerated Constant/1 -> Data Store Write1/1
  Constant1/1 -> Data Store Write2/1

== system SF007A_SysFricLrng/SysFricLrng/SetFricData ==
  note: Set Ram Block Status for 'FricLrngData' moved to Init
  note: update NVM
  FricOffs : Inport
  BasLineFric : Inport  Port=2
  VehLrndFric : Inport  Port=3
  Hys : Inport  Port=4
  RngCntr : Inport  Port=5
  function : TriggerPort  TriggerType=function-call
  CopyRight2 : Subsystem  Description=|  mask(Copyright Information){none=on}
      | Copyright info block.                                               
      |                                                                     
      | Place copyright information at the top of every subsystem in design.
      mask prompts: none "No parameters"
      mask help: Place copyright information at the top of every subsystem in design.
      mask Display:
      | NxtrConf = 'Nexteer Confidential';
      | 
      | sys = bdroot; %handle for the current model ("system")
      | first = get_param(sys,'Created');
      | first = first(end-3:end);  %year is last four digits
      | 
      | last = get_param(sys,'LastModifiedDate');
      | if isempty(last)
      |     last = datestr(now,'yyyy');
      | else
      |     last = last(end-3:end);
      | end
      | 
      | if strcmp(first,last)
      |     fprintf('%s -- Copyright %s Nexteer',NxtrConf,first)
      | else
      |     fprintf('%s -- %s%s- %s Nexteer',NxtrConf,char(169),first,last)
      | end
  Data Store Write3 : DataStoreWrite  DataStoreName=FricLrngData  DataStoreElements=FricLrngData.FricOffs#FricLrngData.BasLineFric(:,:)#FricLrngData.VehLrndFric(:,:)#FricLrngData.Hys(:,:)#FricLrngData.RngCntr(:,:)
  wires:
  Hys/1 -> Data Store Write3/4
  FricOffs/1 -> Data Store Write3/1
  BasLineFric/1 -> Data Store Write3/2
  VehLrndFric/1 -> Data Store Write3/3
  RngCntr/1 -> Data Store Write3/5

== system SF007A_SysFricLrng/SysFricLrng/SetFricLrngData ==
  note: Set Ram Block Status for 'FricLrngData' moved to Init
  note: update NVM
  FricLrngEna : Inport
  FricLrngOffsOutpEna : Inport  Port=2
  FricLrngOperMod : Inport  Port=3
  EolFric : Inport  Port=4
  function : TriggerPort  TriggerType=function-call
  Constant1 : Constant  Value=true  OutDataTypeStr=boolean
      settings: AttributesFormatString=%<OutDataTypeStr>
  CopyRight2 : Subsystem  Description=|  mask(Copyright Information){none=on}
      | Copyright info block.                                               
      |                                                                     
      | Place copyright information at the top of every subsystem in design.
      mask prompts: none "No parameters"
      mask help: Place copyright information at the top of every subsystem in design.
      mask Display:
      | NxtrConf = 'Nexteer Confidential';
      | 
      | sys = bdroot; %handle for the current model ("system")
      | first = get_param(sys,'Created');
      | first = first(end-3:end);  %year is last four digits
      | 
      | last = get_param(sys,'LastModifiedDate');
      | if isempty(last)
      |     last = datestr(now,'yyyy');
      | else
      |     last = last(end-3:end);
      | end
      | 
      | if strcmp(first,last)
      |     fprintf('%s -- Copyright %s Nexteer',NxtrConf,first)
      | else
      |     fprintf('%s -- %s%s- %s Nexteer',NxtrConf,char(169),first,last)
      | end
  Data Store Write : DataStoreWrite  DataStoreName=FricLrngOperModPrev
  Data Store Write1 : DataStoreWrite  DataStoreName=FricLrngData  DataStoreElements=FricLrngData.SysFricLrngOperMod
  Data Store Write3 : DataStoreWrite  DataStoreName=FricNonLrngData  DataStoreElements=FricNonLrngData.EnaFricLrng#FricNonLrngData.EnaFricOffsOutp#FricNonLrngData.EolFric
  Set Ram Block Status1 : NxtrNvM/Set Ram Block Status  FuncName=Set Ram Block Status  NvMBlockName=FricNonLrngData  VoidFuncRtn=on  BlockChanged_DSN=NvMSRBS_BlockChanged  Return_DSN=NvMSRBS_Return
      settings: AttributesFormatString=%<FuncName>
  wires:
  Constant1/1 -> Set Ram Block Status1/1
  FricLrngOperMod/1 -> Data Store Write/1, Data Store Write1/1
  FricLrngEna/1 -> Data Store Write3/1
  FricLrngOffsOutpEna/1 -> Data Store Write3/2
  EolFric/1 -> Data Store Write3/3

== system SF007A_SysFricLrng/SysFricLrng/SetFricOffsOutpDi ==
  FricOffsOutpDi : Inport
  function : TriggerPort  TriggerType=function-call
  CopyRight2 : Subsystem  Description=|  mask(Copyright Information){none=on}
      | Copyright info block.                                               
      |                                                                     
      | Place copyright information at the top of every subsystem in design.
      mask prompts: none "No parameters"
      mask help: Place copyright information at the top of every subsystem in design.
      mask Display:
      | NxtrConf = 'Nexteer Confidential';
      | 
      | sys = bdroot; %handle for the current model ("system")
      | first = get_param(sys,'Created');
      | first = first(end-3:end);  %year is last four digits
      | 
      | last = get_param(sys,'LastModifiedDate');
      | if isempty(last)
      |     last = datestr(now,'yyyy');
      | else
      |     last = last(end-3:end);
      | end
      | 
      | if strcmp(first,last)
      |     fprintf('%s -- Copyright %s Nexteer',NxtrConf,first)
      | else
      |     fprintf('%s -- %s%s- %s Nexteer',NxtrConf,char(169),first,last)
      | end
  Data Store Write : DataStoreWrite  DataStoreName=FricOffsOutpDi
  wires:
  FricOffsOutpDi/1 -> Data Store Write/1

== system SF007A_SysFricLrng/SysFricLrng/SysFricLrngInit1 ==
  note: Note: Removed comments as per anomaly fix to prevent confusion
  function : TriggerPort  TriggerType=function-call
  AssiMechTLpFil : Fil/FilLpInit  Ic=0  Ts=ARCHGLBPRM_10MILLISEC_SEC_F32  Freq=SysFricLrngDataPrepLpFilFrq  StVar=AssiMechTLpFil
  AvrgFricLpFil1 : Fil/FilLpInit  Ic=0  Ts=ARCHGLBPRM_10MILLISEC_SEC_F32  Freq=SysFricLrngAvrgFricFrq  StVar=AvrgFricLpFil1
  AvrgFricLpFil2 : Fil/FilLpInit  Ic=0  Ts=ARCHGLBPRM_10MILLISEC_SEC_F32  Freq=SysFricLrngAvrgFricFrq  StVar=AvrgFricLpFil2
  AvrgFricLpFil3 : Fil/FilLpInit  Ic=0  Ts=ARCHGLBPRM_10MILLISEC_SEC_F32  Freq=SysFricLrngAvrgFricFrq  StVar=AvrgFricLpFil3
  AvrgFricLpFil4 : Fil/FilLpInit  Ic=0  Ts=ARCHGLBPRM_10MILLISEC_SEC_F32  Freq=SysFricLrngAvrgFricFrq  StVar=AvrgFricLpFil4
  ColTqLpFil : Fil/FilLpInit  Ic=0  Ts=ARCHGLBPRM_10MILLISEC_SEC_F32  Freq=SysFricLrngDataPrepLpFilFrq  StVar=ColTqLpFil
  Constant : Constant  Value=VEHSPDPTNUM1_ULS_U08
  Constant1 : Constant  Value=true  OutDataTypeStr=boolean
      settings: AttributesFormatString=%<OutDataTypeStr>
  CopyRight2 : Subsystem  Description=|  mask(Copyright Information){none=on}
      | Copyright info block.                                               
      |                                                                     
      | Place copyright information at the top of every subsystem in design.
      mask prompts: none "No parameters"
      mask help: Place copyright information at the top of every subsystem in design.
      mask Display:
      | NxtrConf = 'Nexteer Confidential';
      | 
      | sys = bdroot; %handle for the current model ("system")
      | first = get_param(sys,'Created');
      | if(isempty(first))
      |     first = datestr(now,'yyyy');
      | else
      |     first = first(end-3:end);  %year is last four digits
      | end
      | 
      | last = get_param(sys,'LastModifiedDate');
      | if isempty(last)
      |     last = datestr(now,'yyyy');
      | else
      |     last = last(end-3:end);
      | end
      | 
      | if strcmp(first,last)
      |     fprintf('%s -- Copyright %s Nexteer',NxtrConf,first)
      | else
      |     fprintf('%s -- %s%s- %s Nexteer',NxtrConf,char(169),first,last)
      | end
  Data Store Read : DataStoreRead  DataStoreName=FricLrngData  DataStoreElements=FricLrngData.SysFricLrngOperMod
  Data Store Read1 : DataStoreRead  DataStoreName=FricLrngData  DataStoreElements=FricLrngData.FricOffs
  Data Store Write : DataStoreWrite  DataStoreName=FricLrngOperModPrev
  Data Store Write1 : DataStoreWrite  DataStoreName=RefTmrLrngConstr
  Data Store Write2 : DataStoreWrite  DataStoreName=RefTmrNtc
  FricChgLpFil : Fil/FilLpInit  Ic=0  Ts=ARCHGLBPRM_10MILLISEC_SEC_F32  Freq=SysFricLrngFricOffsLpFilFrq  StVar=FricChgLpFil
  GetRefTmr100MicroSec32bit : Subsystem
  GetRefTmr100MicroSec32bit1 : Subsystem
  HwAgAuthyLpFil : Fil/FilLpInit  Ic=0  Ts=ARCHGLBPRM_10MILLISEC_SEC_F32  Freq=SysFricLrngDataPrepLpFilFrq  StVar=HwAgAuthyLpFil
  HwAgLpFil : Fil/FilLpInit  Ic=0  Ts=ARCHGLBPRM_10MILLISEC_SEC_F32  Freq=SysFricLrngDataPrepLpFilFrq  StVar=HwAgLpFil
  HwVelLpFil : Fil/FilLpInit  Ic=0  Ts=ARCHGLBPRM_10MILLISEC_SEC_F32  Freq=SysFricLrngDataPrepLpFilFrq  StVar=HwVelLpFil
  Initialization : Subsystem  RequirementInfo={} %GIDa_91d738c7_e712_4f5c_81ea_e86a6bba312a  Priority=1  TreatAsAtomicUnit=on
  LatALpFil : Fil/FilLpInit  Ic=0  Ts=ARCHGLBPRM_10MILLISEC_SEC_F32  Freq=SysFricLrngDataPrepLpFilFrq  StVar=LatALpFil
  Set Ram Block Status : NxtrNvM/Set Ram Block Status  FuncName=Set Ram Block Status  NvMBlockName=FricLrngData  VoidFuncRtn=on  BlockChanged_DSN=NvMSRBS_BlockChanged  Return_DSN=NvMSRBS_Return
      settings: AttributesFormatString=%<FuncName>
  VehSpdLpFil : Fil/FilLpInit  Ic=0  Ts=ARCHGLBPRM_10MILLISEC_SEC_F32  Freq=SysFricLrngDataPrepLpFilFrq  StVar=VehSpdLpFil
  SysFricOffs : Outport
  wires:
  Data Store Read/1 -> Data Store Write/1
  GetRefTmr100MicroSec32bit/1(RefTmr) -> Data Store Write1/1
  Constant/1 -> Initialization/1(VEHSPDPTNUM1_ULS_U08)
  Data Store Read1/1 -> SysFricOffs/1
  GetRefTmr100MicroSec32bit1/1(RefTmr) -> Data Store Write2/1
  Constant1/1 -> Set Ram Block Status/1
